simulink model "6DoF_V8_2024a_FULLY_WORKING_FG"  (R2024b)
settings: Solver=ode45  StartTime=0.0  StopTime=500  FixedStep=.01  MaxStep=.004  RelTol=1e-5  EnableMultiTasking=on
values from neighbouring files (symbols this model uses):
  ac = [0 0 0]    [Geom_6dof_V4_WITH_MAP.m]
  b = 33.4    [Geom_6dof_V4_WITH_MAP.m]
  bankrange = linspace(-pi,pi,100)    [Geom_6dof_V4_WITH_MAP.m]
  cbar = 5.7    [Geom_6dof_V4_WITH_MAP.m]
  cda2 = 0.33    [Geom_6dof_V4_WITH_MAP.m]
  cdo = 0.05    [Geom_6dof_V4_WITH_MAP.m]
  cg = [0 0 0]    [Geom_6dof_V4_WITH_MAP.m]
  cla = 4.44    [Geom_6dof_V4_WITH_MAP.m]
  cladot = 0    [Geom_6dof_V4_WITH_MAP.m]
  clb = -0.074    [Geom_6dof_V4_WITH_MAP.m]
  clda = -0.134    [Geom_6dof_V4_WITH_MAP.m]
  clde = 0.355    [Geom_6dof_V4_WITH_MAP.m]
  cldr = 0.107    [Geom_6dof_V4_WITH_MAP.m]
  clo = 0.41    [Geom_6dof_V4_WITH_MAP.m]
  clp = -0.410    (= -0.41)    [Geom_6dof_V4_WITH_MAP.m]
  clq = 3.8    [Geom_6dof_V4_WITH_MAP.m]
  clr = 0.107    [Geom_6dof_V4_WITH_MAP.m]
  cma = -0.683    [Geom_6dof_V4_WITH_MAP.m]
  cmadot = -4.36    [Geom_6dof_V4_WITH_MAP.m]
  cmde = -0.923    [Geom_6dof_V4_WITH_MAP.m]
  cmq = -9.96    [Geom_6dof_V4_WITH_MAP.m]
  cnb = 0.071    [Geom_6dof_V4_WITH_MAP.m]
  cnda = -0.0035    [Geom_6dof_V4_WITH_MAP.m]
  cndr = -0.072    [Geom_6dof_V4_WITH_MAP.m]
  cnp = -0.0575    [Geom_6dof_V4_WITH_MAP.m]
  cnr = -0.125    [Geom_6dof_V4_WITH_MAP.m]
  cyb = -0.564    [Geom_6dof_V4_WITH_MAP.m]
  cydr = 0.157    [Geom_6dof_V4_WITH_MAP.m]
  eng = [0 0 0]    [Geom_6dof_V4_WITH_MAP.m]
  initalt = 5000    [Geom_6dof_V4_WITH_MAP.m]
  initbank = 0    [Geom_6dof_V4_WITH_MAP.m]
  initeast = 0    [Geom_6dof_V4_WITH_MAP.m]
  inithead = 0    [Geom_6dof_V4_WITH_MAP.m]
  initnorth = 0    [Geom_6dof_V4_WITH_MAP.m]
  initp = 0    [Geom_6dof_V4_WITH_MAP.m]
  initpitch = initw/initu    (= -0.0287187462721)    [Geom_6dof_V4_WITH_MAP.m]
  initq = 0    [Geom_6dof_V4_WITH_MAP.m]
  initr = 0    [Geom_6dof_V4_WITH_MAP.m]
  initu = 226.333    [Geom_6dof_V4_WITH_MAP.m]
  initv = 0    [Geom_6dof_V4_WITH_MAP.m]
  initw = -6.5    [Geom_6dof_V4_WITH_MAP.m]
  jx = 1048    [Geom_6dof_V4_WITH_MAP.m]
  jxz = 0    [Geom_6dof_V4_WITH_MAP.m]
  jy = 3000    [Geom_6dof_V4_WITH_MAP.m]
  jz = 3500    [Geom_6dof_V4_WITH_MAP.m]
  sw = 184    [Geom_6dof_V4_WITH_MAP.m]
  weight = 2750    [Geom_6dof_V4_WITH_MAP.m]
  WP1 = [10000 10000 5000]    [Geom_6dof_V4_WITH_MAP.m]
  WP2 = [-10000 0 5500]    [Geom_6dof_V4_WITH_MAP.m]
  WP3 = [0 -10000 4500]    [Geom_6dof_V4_WITH_MAP.m]
libraries: slpidlib x10, simulink_extras x5, aerolibfltsims x2, aerolibanimutils x1, dspswit3 x1
(part 1 of 2)
settings Model: Creator=andersop  LastModifiedBy=Owner
settings SolverCC: InitialStep=.004  AlgebraicLoopSolver=TrustRegion
settings DataIOCC: LimitDataPoints=on  SaveFormat=Array  SignalLoggingSaveFormat=ModelDataLogs  SaveState=on  ReturnWorkspaceOutputs=off  SignalLoggingName=sigsOut
settings OptimizationCC: ExpressionDepthLimit=2147483647  InitFltsAndDblsToZero=on  LifeSpan=inf
settings DebuggingCC: SaveWithParameterizedLinksMsg=none  UnderspecifiedInitializationDetection=Classic  MergeDetectMultiDrivingBlocksExec=none  SignalResolutionControl=TryResolveAllWithWarning  MultiTaskDSMMsg=warning  MultiTaskCondExecSysMsg=none  FcnCallInpInsideContextMsg=warning  UnconnectedInputMsg=warning  UnconnectedOutputMsg=warning  UnconnectedLineMsg=warning  StateNameClashWarn=warning  SFUnexpectedBacktrackingDiag=warning  SFNoUnconditionalDefaultTransitionDiag=warning  SFExecutionAtInitializationDiag=none  ArithmeticOperatorsInVariantConditions=warning
settings HardwareCC: ProdBitPerPointer=32  ProdBitPerSizeT=32  ProdBitPerPtrDiffT=32  ProdLargestAtomicFloat=None  ProdIntDivRoundTo=Undefined  ProdEndianess=Unspecified  ProdWordSize=32  ProdHWDeviceType=32-bit Generic  TargetUnknown=on
settings ModelReferenceCC: PropagateSignalLabelsOutOfModel=off
settings SFSimCC: SimUseLocalCustomCode=off  CustomCodeUndefinedFunction=UseInterfaceOnly
settings RTWCC: RTWUseLocalCustomCode=off  GPUComputeCapability=3.5
settings CodeAppCC: StateflowObjectComments=on
settings GRTTargetCC: TargetFcnLib=ansi_tfl_tmw.mat  TargetLangStandard=C89/C90 (ANSI)  ModelReferenceCompliant=off  CombineOutputUpdateFcns=off  MatFileLogging=off  GRTInterface=on
settings ConfigComp: CovMetricSettings=dw  CovSaveCumulativeToWorkspaceVar=on  CovSaveSingleToWorkspaceVar=on  CovExternalEMLEnable=off

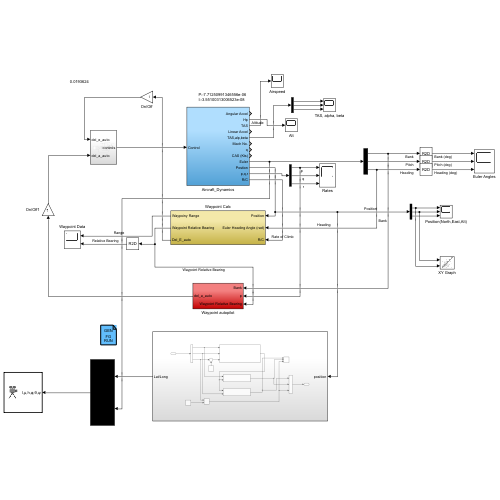
[thumbnail: Simulink's stored preview of the top-level diagram]
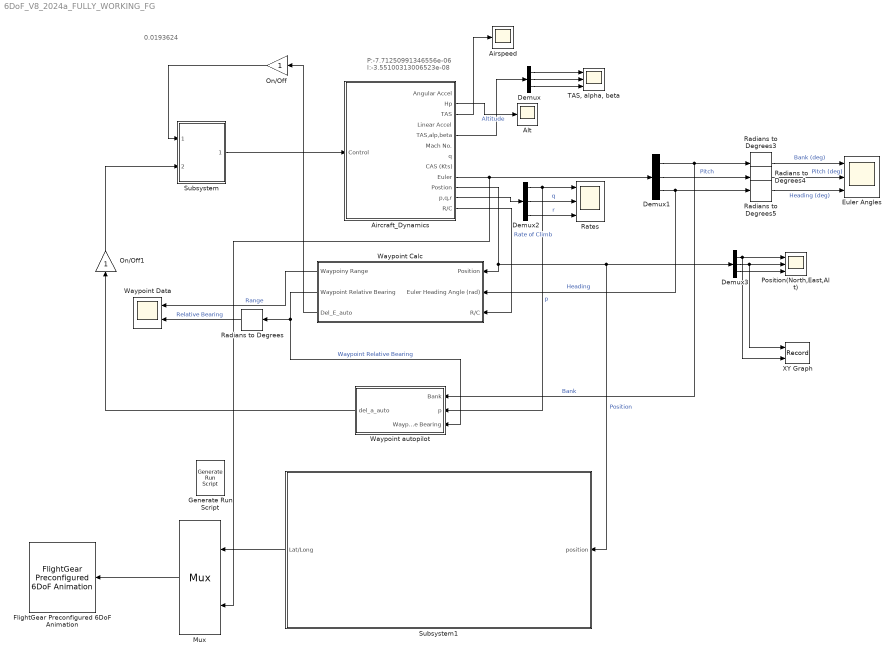
== system 6DoF_V8_2024a_FULLY_WORKING_FG ==
  note: P:-7.71250991346556e-06
      | I:-3.55100313006523e-08
  note: 0.0193624
  Aircraft_Dynamics : Subsystem
  Airspeed : Scope
  Alt : Scope
  Demux{,1..3} (4 alike) : Demux  Outputs=3
  Euler Angles : Scope  NumInputPorts=3
  FlightGear Preconfigured 6DoF Animation : aerolibfltsims/FlightGear Preconfigured 6DoF Animation  xFlightGearVersion=v2019.1  DestinationIpAddress=127.0.0.1  DestinationPort=5502  SampleTime=1/30  packetVersion=24
  Generate Run Script : aerolibfltsims/Generate Run Script  Architecture=Win64  dataFlow=Send  GeometryModelName=c172p  AirportId=KSFO  RunwayId=10L  InitialAltitude=5000  InitialHeading=0  OffsetDistance=4.72  OffsetAzimuth=0  InstallScenery=off  DisableShaders=off  OriginAddress=127.0.0.1  DestinationPort=5502  OriginPort=5505  LocalAddress=127.0.0.1  OutputFileName=runfg.bat  FlightGearBaseDirectory=C:\Program Files\FlightGear 2020.3
  Mux : Mux  Inputs=2
  On/Off : Gain
  On/Off1 : Gain
  Position(North,East,Alt) : Scope  NumInputPorts=3
  Radians to Degrees{,3..5} (4 alike) : simulink_extras/Transformations/Radians to Degrees
  Rates : Scope  NumInputPorts=3
  Subsystem : Subsystem
  Subsystem1 : Subsystem
  "TAS, alpha, beta" : Scope  NumInputPorts=3
  Waypoint Calc : Subsystem
  Waypoint Data : Scope  NumInputPorts=2
  Waypoint autopilot : Subsystem
  XY Graph : Record  FileSettingsInternal="{\"entries\":[{\"content\":{\"excelSettings\":{\"content\":{},\"type\":\"Streamout.ExcelSettings\"}},\"type\":\"Streamout.FileSettingStorage\",\"uuid\":\"\"}],\"packageUris\":[\"http:\\/\\/schema.mathworks.com\\/mf0\\/streamout_blocks\\/R2020a\"],\"version\":\"1.0\"}"  Layout=[1 1]  SignalsInternal="{\"entries\":[{\"content\":{\"signals\":[{\"content\":{\"blockPath\":[],\"dimensions\":[1],\"domain\":\"\",\"lineColor\":\"#a2142f\",\"plots\":[ 1 ],\"port\":1,\"sid\":[\"\"],\"signalID\":1,\"signalName\":\"Demux3:2\"},\"type\":\"RecordBlkView.Signal\",\"uuid\":\"\"},{\"content\":{\"blockPath\":[],\"dimensions\":[1],\"domain\":\"\",\"lineColor\":\"#139fff\",\"plots\":[ 1 ],\"port\":2,\"sid\":[\"\"],\"signalID\":2,\"signalName\":\"Demux3:1\"},\"type\":\"RecordBlkView.Signal\",\"uuid\":\"\"}]},\"type\":\"RecordBlkView.InputSignals\",\"uuid\":\"\"}],\"packageUris\":[\"http:\\/\\/schema.mathworks.com\\/mf0\\/streamout_blocks\\/R2020a\"],\"version\":\"1.0\"}"  VisualizationBindings="{\"xyplotplugin\":{\"info\":[{\"series\":[{\"bindingParametersList\":[{\"parameter\":\"X-Axis\",\"signalID\":1,\"signalName\":\"Demux3:2\"},{\"parameter\":\"Y-Axis\",\"signalID\":2,\"signalName\":\"Demux3:1\"}],\"seriesID\":0}],\"subplotID\":1}]}}"  CompatibilityTag=XY
  wires:
  Aircraft_Dynamics/9(Euler) -> Mux/2, Demux1/1
  Aircraft_Dynamics/3(TAS) -> Airspeed/1
  Aircraft_Dynamics/5(TAS,alp,beta) -> Demux/1
  Demux1/1 -> Waypoint autopilot/1(Bank), Radians to Degrees3/1  "Bank"
  Demux1/2 -> Radians to Degrees4/1  "Pitch"
  Demux1/3 -> Radians to Degrees5/1, Waypoint Calc/2(Euler Heading Angle (rad))  "Heading"
  Demux/1 -> "TAS, alpha, beta"/1
  Demux/2 -> "TAS, alpha, beta"/2
  Demux/3 -> "TAS, alpha, beta"/3
  Demux2/1 -> Rates/1, Waypoint autopilot/2(p)  "p"
  Demux2/2 -> Rates/2  "q"
  Demux2/3 -> Rates/3  "r"
  Aircraft_Dynamics/11(p,q,r) -> Demux2/1
  Aircraft_Dynamics/12(R/C) -> Waypoint Calc/3(R/C)  "Rate of Climb"
  Aircraft_Dynamics/10(Postion) -> Subsystem1/1(position), Demux3/1, Waypoint Calc/1(Position)  "Position"
  Demux3/1 -> XY Graph/2, Position(North,East,Alt)/1
  Demux3/2 -> XY Graph/1, Position(North,East,Alt)/2
  Demux3/3 -> Position(North,East,Alt)/3
  Waypoint Calc/1(Waypoiny Range) -> Waypoint Data/1  "Range"
  Waypoint Calc/2(Waypoint Relative Bearing) -> Radians to Degrees/1, Waypoint autopilot/3(Waypoint Relative Bearing)  "Waypoint Relative Bearing"
  Radians to Degrees/1 -> Waypoint Data/2  "Relative Bearing"
  Waypoint Calc/3(Del_E_auto) -> On/Off/1
  Radians to Degrees3/1 -> Euler Angles/1  "Bank (deg)"
  Radians to Degrees4/1 -> Euler Angles/2  "Pitch (deg)"
  Radians to Degrees5/1 -> Euler Angles/3  "Heading (deg)"
  Waypoint autopilot/1(del_a_auto) -> On/Off1/1
  Aircraft_Dynamics/2(Hp) -> Alt/1  "Altitude"
  Subsystem/1(controls) -> Aircraft_Dynamics/1(Control)
  On/Off/1 -> Subsystem/1(del_e_auto)
  On/Off1/1 -> Subsystem/2(del_a_auto)
  Subsystem1/1(Lat/Long) -> Mux/1
  Mux/1 -> FlightGear Preconfigured 6DoF Animation/1

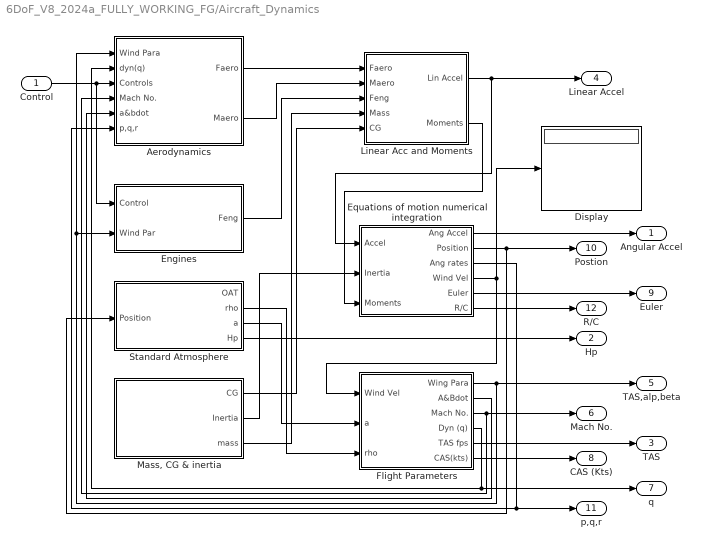
== system 6DoF_V8_2024a_FULLY_WORKING_FG/Aircraft_Dynamics ==
  Control : Inport
  Aerodynamics : Subsystem
  Display : Display
  Engines : Subsystem
  "Equations of motion numerical integration " : Subsystem
  Flight Parameters : Subsystem
  Linear Acc and Moments : Subsystem
  "Mass, CG & inertia" : Subsystem
  Standard Atmosphere : Subsystem
  Angular Accel : Outport
  Hp : Outport  Port=2
  TAS : Outport  Port=3
  Linear Accel : Outport  Port=4
  TAS,alp,beta : Outport  Port=5
  Mach No. : Outport  Port=6
  q : Outport  Port=7
  CAS (Kts) : Outport  Port=8
  Euler : Outport  Port=9
  Postion : Outport  Port=10
  p,q,r : Outport  Port=11
  R/C : Outport  Port=12
  wires:
  Aerodynamics/1(Faero) -> Linear Acc and Moments/1(Faero)
  Aerodynamics/2(Maero) -> Linear Acc and Moments/2(Maero)
  Control/1 -> Aerodynamics/3(Controls), Engines/1(Control)
  Engines/1(Feng) -> Linear Acc and Moments/3(Feng)
  "Mass, CG & inertia"/1(CG) -> Linear Acc and Moments/5(CG)
  "Mass, CG & inertia"/2(Inertia) -> "Equations of motion numerical integration "/2(Inertia)
  Linear Acc and Moments/1(Lin Accel) -> "Equations of motion numerical integration "/1(Accel), Linear Accel/1
  Linear Acc and Moments/2(Moments) -> "Equations of motion numerical integration "/3(Moments)
  "Equations of motion numerical integration "/3(Ang rates) -> Aerodynamics/6(p,q,r), p,q,r/1
  "Equations of motion numerical integration "/4(Wind Vel) -> Flight Parameters/1(Wind Vel), Display/1
  Flight Parameters/1(Wing Para) -> TAS,alp,beta/1, Aerodynamics/1(Wind Para), Engines/2(Wind Par)
  Flight Parameters/4(Dyn (q)) -> Aerodynamics/2(dyn(q)), q/1
  Flight Parameters/3(Mach No.) -> Mach No./1, Aerodynamics/4(Mach No.)
  Flight Parameters/2(A&Bdot) -> Aerodynamics/5(a&bdot)
  "Equations of motion numerical integration "/2(Position) -> Standard Atmosphere/1(Position), Postion/1
  "Equations of motion numerical integration "/1(Ang Accel) -> Angular Accel/1
  Standard Atmosphere/4(Hp) -> Hp/1
  Flight Parameters/5(TAS fps) -> TAS/1
  Flight Parameters/6(CAS(kts)) -> CAS (Kts)/1
  "Equations of motion numerical integration "/5(Euler) -> Euler/1
  Standard Atmosphere/3(a) -> Flight Parameters/2(a)
  Standard Atmosphere/2(rho) -> Flight Parameters/3(rho)
  "Mass, CG & inertia"/3(mass) -> Linear Acc and Moments/4(Mass)
  "Equations of motion numerical integration "/6(R/C) -> R/C/1

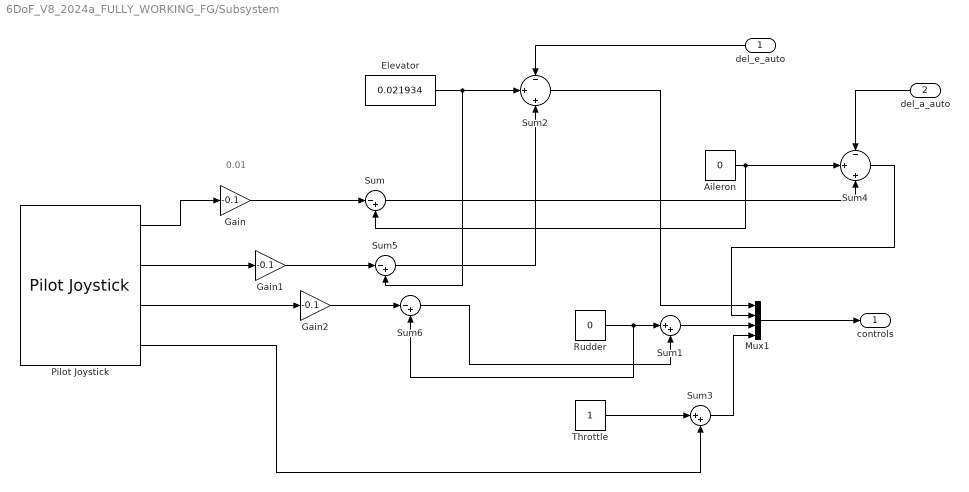
== system 6DoF_V8_2024a_FULLY_WORKING_FG/Subsystem ==
  note: 0.01
  del_e_auto : Inport
  del_a_auto : Inport  Port=2
  Aileron : Constant  Value=0
  Elevator : Constant  Value=0.021934
  Gain : Gain  Gain=-0.1
  Gain1 : Gain  Gain=-0.1
  Gain2 : Gain  Gain=-0.1
  Mux1 : Mux
  Pilot Joystick : aerolibanimutils/Pilot Joystick  JoystickID=Joystick1  OutputConfiguration=FourAxis  SampleTime=1/30
  Rudder : Constant  Value=0
  Sum : Sum  Inputs=|-+
  Sum1 : Sum  Inputs=|++
  Sum2 : Sum  Inputs=-|+|+
  Sum3 : Sum  Inputs=|++
  Sum4 : Sum  Inputs=-|+|+
  Sum5 : Sum  Inputs=|-+
  Sum6 : Sum  Inputs=|-+
  Throttle : Constant
  controls : Outport
  wires:
  Elevator/1 -> Sum2/2, Sum5/2
  Pilot Joystick/1 -> Gain/1
  Gain1/1 -> Sum5/1
  Pilot Joystick/3 -> Gain2/1
  Sum2/1 -> Mux1/1
  Sum4/1 -> Mux1/2
  Pilot Joystick/2 -> Gain1/1
  Gain2/1 -> Sum6/1
  Sum5/1 -> Sum2/3
  Gain/1 -> Sum/1
  Mux1/1 -> controls/1
  del_e_auto/1 -> Sum2/1
  Aileron/1 -> Sum4/2, Sum/2
  Sum/1 -> Sum4/3
  del_a_auto/1 -> Sum4/1
  Rudder/1 -> Sum6/2, Sum1/1
  Sum6/1 -> Sum1/2
  Sum1/1 -> Mux1/3
  Throttle/1 -> Sum3/1
  Pilot Joystick/4 -> Sum3/2
  Sum3/1 -> Mux1/4

== system 6DoF_V8_2024a_FULLY_WORKING_FG/Subsystem1 ==
  position : Inport
  Demux : Demux  Outputs=3
  Earth : Constant  Value=20925000
  MATLAB Function : MATLAB Function  TreatAsAtomicUnit=on
  MATLAB Function1 : MATLAB Function  TreatAsAtomicUnit=on
  Mux : Mux  Inputs=3
  "NED to LAT/LONG " : Subsystem
  Product : Product
  Scope : Scope  NumInputPorts=3
  Sum : Sum  Inputs=|++
  ft - m conversion : Constant  Value=0.3048
  Lat/Long : Outport
  wires:
  Mux/1 -> Lat/Long/1
  Demux/3 -> Product/1, Sum/1
  Demux/1 -> MATLAB Function/1(N), "NED to LAT/LONG "/1(N)
  "NED to LAT/LONG "/1(r) -> MATLAB Function1/1(r), MATLAB Function/2(r)
  MATLAB Function/1(Lat) -> Mux/2, Scope/2
  Demux/2 -> MATLAB Function1/2(E), "NED to LAT/LONG "/2(E)
  Sum/1 -> "NED to LAT/LONG "/3(D)
  position/1 -> Demux/1
  Earth/1 -> Sum/2
  MATLAB Function1/1(Long) -> Mux/1, Scope/1
  Product/1 -> Mux/3, Scope/3
  ft - m conversion/1 -> Product/2

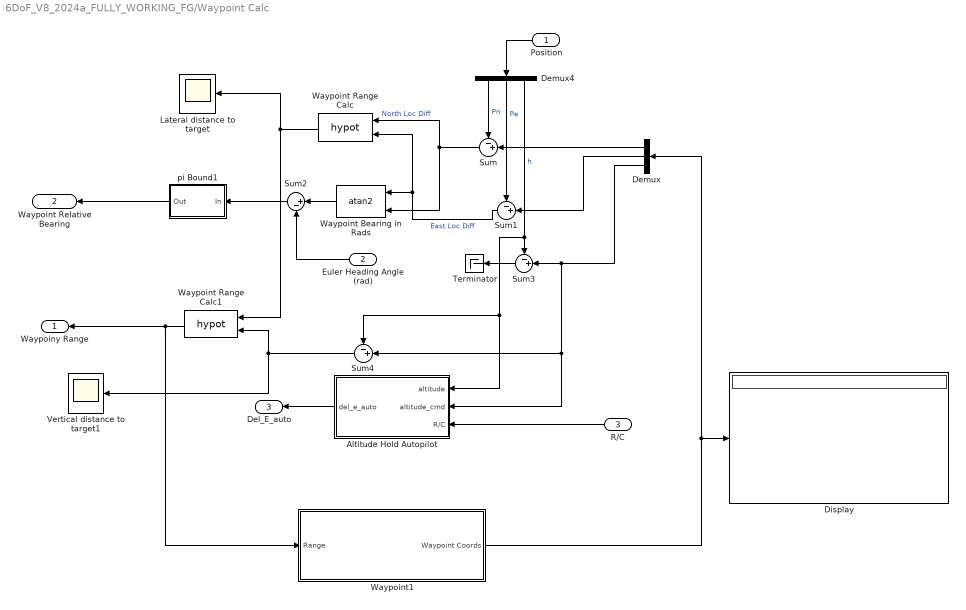
== system 6DoF_V8_2024a_FULLY_WORKING_FG/Waypoint Calc ==
  Position : Inport
  Euler Heading Angle (rad) : Inport  Port=2
  R/C : Inport  Port=3
  Altitude Hold Autopilot : Subsystem
  Demux : Demux  Outputs=3
  Demux4 : Demux  Outputs=3
  Display : Display
  Lateral distance to target : Scope
  Sum{,1,3..4} (4 alike) : Sum  Inputs=-+|
  Sum2 : Sum  Inputs=|+-
  Terminator : Terminator
  Vertical distance to target1 : Scope
  Waypoint Bearing in Rads : Trigonometry  Operator=atan2
  Waypoint Range Calc : Math  Operator=hypot
  Waypoint Range Calc1 : Math  Operator=hypot
  Waypoint1 : Subsystem
  pi Bound1 : Subsystem  mask(pi bound){}
      mask help: Bounds the input angle to [-pi, pi]. When -pi bound is exceeded the output wraps back to pi; when the pi bound is exceeded the output wraps back to -pi.
      mask Help:
      | Bounds the input angle to [-pi, pi]. When -pi bound is exceeded the output wraps back to pi; when the pi bound is exceeded the output wraps back to -pi.
      | <P><B>Input:</B> any angle in radians, from -Inf to Inf;</P>
      | <P><B>Output:</B> an angle in radians between -pi and pi.</P>
  Waypoiny Range : Outport
  Waypoint Relative Bearing : Outport  Port=2
  Del_E_auto : Outport  Port=3
  wires:
  Demux4/2 -> Sum1/1  "Pe"
  Sum/1 -> Waypoint Bearing in Rads/2, Waypoint Range Calc/1  "North Loc Diff"
  Demux4/3 -> Sum4/1, Altitude Hold Autopilot/1(altitude), Sum3/1  "h"
  Sum1/1 -> Waypoint Bearing in Rads/1, Waypoint Range Calc/2  "East Loc Diff"
  Sum3/1 -> Terminator/1
  Demux4/1 -> Sum/1  "Pn"
  Position/1 -> Demux4/1
  Waypoint Range Calc/1 -> Lateral distance to target/1, Waypoint Range Calc1/1
  Euler Heading Angle (rad)/1 -> Sum2/2
  Waypoint Bearing in Rads/1 -> Sum2/1
  Sum2/1 -> pi Bound1/1(In)
  pi Bound1/1(Out) -> Waypoint Relative Bearing/1
  Demux/1 -> Sum/2
  Demux/2 -> Sum1/2
  Demux/3 -> Altitude Hold Autopilot/2(altitude_cmd), Sum4/2, Sum3/2
  R/C/1 -> Altitude Hold Autopilot/3(R/C)
  Sum4/1 -> Vertical distance to target1/1, Waypoint Range Calc1/2
  Waypoint Range Calc1/1 -> Waypoint1/1(Range), Waypoiny Range/1
  Altitude Hold Autopilot/1(del_e_auto) -> Del_E_auto/1
  Waypoint1/1(Waypoint Coords) -> Demux/1, Display/1

== system 6DoF_V8_2024a_FULLY_WORKING_FG/Waypoint autopilot ==
  Bank : Inport
  p : Inport  Port=2
  Waypoint Relative Bearing : Inport  Port=3
  1 : slpidlib/PID Controller  Controller=PI  Form=Parallel  TimeDomain=Continuous-time  UseExternalTs=off  SampleTime=-1  IntegratorMethod=Forward Euler  FilterMethod=Forward Euler  ControllerParametersSource=internal  P=0.0442231432191756  I=0.000555878552542947  UseKiTs=off  D=-0.00015961532293143  UseExternalDerivativeSource=off  N=22.9108316729658  UseFilter=on  TunerSelectOption=Transfer Function Based (PID Tuner App)  InitialConditionSource=internal  InitialConditionForIntegrator=0  InitialConditionForFilter=0  DifferentiatorICPrevScaledInput=0  ExternalReset=none  TrackingMode=off  Kt=1  LimitOutput=off  SatLimitsSource=internal  UpperSaturationLimit=inf  LowerSaturationLimit=-inf  LinearizeAsGain=on  AntiWindupMode=none  Kb=1  LimitIntegrator=off  UpperIntegratorSaturationLimit=inf  LowerIntegratorSaturationLimit=-inf  POutMin=[]  POutMax=[]  IOutMin=[]  IOutMax=[]  DOutMin=[]  DOutMax=[]  NOutMin=[]  NOutMax=[]  SumOutMin=[]  SumOutMax=[]  SaturationOutMin=[]  SaturationOutMax=[]  PParamMin=[]  PParamMax=[]  IParamMin=[]  IParamMax=[]  DParamMin=[]  DParamMax=[]  NParamMin=[]  NParamMax=[]  KbParamMin=[]  KbParamMax=[]  KtParamMin=[]  KtParamMax=[]  KbOutMin=[]  KbOutMax=[]  KtOutMin=[]  KtOutMax=[]  IntegratorOutMin=[]  IntegratorOutMax=[]  FilterOutMin=[]  FilterOutMax=[]  SumI1OutMin=[]  SumI1OutMax=[]  SumI2OutMin=[]  SumI2OutMax=[]  SumI3OutMin=[]  SumI3OutMax=[]  SumI4OutMin=[]  SumI4OutMax=[]  SumDOutMin=[]  SumDOutMax=[]  DifferentiatorOutMin=[]  DifferentiatorOutMax=[]  FilterDiffOutCoefMin=[]  FilterDiffOutCoefMax=[]  ReciprocalOutMin=[]  ReciprocalOutMax=[]  SumDenOutMin=[]  SumDenOutMax=[]  SumNumOutMin=[]  SumNumOutMax=[]  DivideOutMin=[]  DivideOutMax=[]  UdiffTsProdOutMin=[]  UdiffTsProdOutMax=[]  NTsProdOutMin=[]  NTsProdOutMax=[]  UintegralTsProdOutMin=[]  UintegralTsProdOutMax=[]  UngainTsProdOutMin=[]  UngainTsProdOutMax=[]  ClampingZeroOutDataTypeStr=Inherit: Inherit via back propagation  ClampingZeroOutMin=[]  ClampingZeroOutMax=[]  FilterDenConstantOutDataTypeStr=Inherit: Inherit via back propagation  FilterDenConstantOutMin=[]  FilterDenConstantOutMax=[]  PCopyOutDataTypeStr=Inherit: Inherit via back propagation  PCopyOutMin=[]  PCopyOutMax=[]  NCopyOutDataTypeStr=Inherit: Inherit via back propagation  NCopyOutMin=[]  NCopyOutMax=[]  IntegratorContinuousStateAttributes=''  IntegratorStateMustResolveToSignalObject=off  IntegratorRTWStateStorageClass=Auto  FilterContinuousStateAttributes=''  FilterStateMustResolveToSignalObject=off  FilterRTWStateStorageClass=Auto  ParallelPVariant=InternalParameters  IdealPVariant=Disabled  IVariant=InternalParameters  DVariant=Disabled  IntegratorVariant=Continuous  SatVariant=Disabled  AWVariant=Passthrough  PCopyVariant=Disabled  TRVariant=Disabled  FdbkBlocksVariant=Forward  IdealPFdbkVariant=Disabled  SatFdbkVariant=Disabled  DerivativeFilterVariant=Disabled  NVariant=Disabled  NCopyVariant=Disabled_SignalSpec  FilterICVariant=Disabled  IntegratorICVariant=InternalICs  ExternalResetVariant=Disabled  TRSumVariant=Passthrough  SumFdbkVariant=Disabled  SumVariant=Sum_PI  TsampFilterVariant=InternalTs  TsampNgainVariant=Passthrough  TsampIntegralVariant=Disabled_SignalSpec  ExternalSaturationOutDataTypeStr=Inherit: Same as second input  DerivativeSourceVariant=Disabled  PreIntVariant=InternalPreInt
  2 : slpidlib/PID Controller  Controller=PI  Form=Parallel  TimeDomain=Continuous-time  UseExternalTs=off  SampleTime=-1  IntegratorMethod=Forward Euler  FilterMethod=Forward Euler  ControllerParametersSource=internal  P=0.0813778181648477  I=0.00542773234625677  UseKiTs=off  D=-0.00015961532293143  UseExternalDerivativeSource=off  N=22.9108316729658  UseFilter=on  TunerSelectOption=Transfer Function Based (PID Tuner App)  InitialConditionSource=internal  InitialConditionForIntegrator=0  InitialConditionForFilter=0  DifferentiatorICPrevScaledInput=0  ExternalReset=none  TrackingMode=off  Kt=1  LimitOutput=off  SatLimitsSource=internal  UpperSaturationLimit=inf  LowerSaturationLimit=-inf  LinearizeAsGain=on  AntiWindupMode=none  Kb=1  LimitIntegrator=off  UpperIntegratorSaturationLimit=inf  LowerIntegratorSaturationLimit=-inf  POutMin=[]  POutMax=[]  IOutMin=[]  IOutMax=[]  DOutMin=[]  DOutMax=[]  NOutMin=[]  NOutMax=[]  SumOutMin=[]  SumOutMax=[]  SaturationOutMin=[]  SaturationOutMax=[]  PParamMin=[]  PParamMax=[]  IParamMin=[]  IParamMax=[]  DParamMin=[]  DParamMax=[]  NParamMin=[]  NParamMax=[]  KbParamMin=[]  KbParamMax=[]  KtParamMin=[]  KtParamMax=[]  KbOutMin=[]  KbOutMax=[]  KtOutMin=[]  KtOutMax=[]  IntegratorOutMin=[]  IntegratorOutMax=[]  FilterOutMin=[]  FilterOutMax=[]  SumI1OutMin=[]  SumI1OutMax=[]  SumI2OutMin=[]  SumI2OutMax=[]  SumI3OutMin=[]  SumI3OutMax=[]  SumI4OutMin=[]  SumI4OutMax=[]  SumDOutMin=[]  SumDOutMax=[]  DifferentiatorOutMin=[]  DifferentiatorOutMax=[]  FilterDiffOutCoefMin=[]  FilterDiffOutCoefMax=[]  ReciprocalOutMin=[]  ReciprocalOutMax=[]  SumDenOutMin=[]  SumDenOutMax=[]  SumNumOutMin=[]  SumNumOutMax=[]  DivideOutMin=[]  DivideOutMax=[]  UdiffTsProdOutMin=[]  UdiffTsProdOutMax=[]  NTsProdOutMin=[]  NTsProdOutMax=[]  UintegralTsProdOutMin=[]  UintegralTsProdOutMax=[]  UngainTsProdOutMin=[]  UngainTsProdOutMax=[]  ClampingZeroOutDataTypeStr=Inherit: Inherit via back propagation  ClampingZeroOutMin=[]  ClampingZeroOutMax=[]  FilterDenConstantOutDataTypeStr=Inherit: Inherit via back propagation  FilterDenConstantOutMin=[]  FilterDenConstantOutMax=[]  PCopyOutDataTypeStr=Inherit: Inherit via back propagation  PCopyOutMin=[]  PCopyOutMax=[]  NCopyOutDataTypeStr=Inherit: Inherit via back propagation  NCopyOutMin=[]  NCopyOutMax=[]  IntegratorContinuousStateAttributes=''  IntegratorStateMustResolveToSignalObject=off  IntegratorRTWStateStorageClass=Auto  FilterContinuousStateAttributes=''  FilterStateMustResolveToSignalObject=off  FilterRTWStateStorageClass=Auto  ParallelPVariant=InternalParameters  IdealPVariant=Disabled  IVariant=InternalParameters  DVariant=Disabled  IntegratorVariant=Continuous  SatVariant=Disabled  AWVariant=Passthrough  PCopyVariant=Disabled  TRVariant=Disabled  FdbkBlocksVariant=Forward  IdealPFdbkVariant=Disabled  SatFdbkVariant=Disabled  DerivativeFilterVariant=Disabled  NVariant=Disabled  NCopyVariant=Disabled_SignalSpec  FilterICVariant=Disabled  IntegratorICVariant=InternalICs  ExternalResetVariant=Disabled  TRSumVariant=Passthrough  SumFdbkVariant=Disabled  SumVariant=Sum_PI  TsampFilterVariant=InternalTs  TsampNgainVariant=Passthrough  TsampIntegralVariant=Disabled_SignalSpec  ExternalSaturationOutDataTypeStr=Inherit: Same as second input  DerivativeSourceVariant=Disabled  PreIntVariant=InternalPreInt
  Bank Err : Scope
  Bearing Lookup1 : Lookup_n-D  NumberOfTableDimensions=1  BreakpointsForDimension1=bankrange  BreakpointsForDimension1Spacing=30  Table=(1.5/pi)*atan(bankrange)  InternalRulePriority=Speed  RndMeth=Simplest
  Del_a : Scope
  Orig : slpidlib/PID Controller  Controller=PI  Form=Parallel  TimeDomain=Continuous-time  UseExternalTs=off  SampleTime=-1  IntegratorMethod=Forward Euler  FilterMethod=Forward Euler  ControllerParametersSource=internal  P=0.0584144917265337 *2.63  I=0.0031457168401691*0.57  UseKiTs=off  D=0  UseExternalDerivativeSource=off  N=100  UseFilter=on  TunerSelectOption=Transfer Function Based (PID Tuner App)  InitialConditionSource=internal  InitialConditionForIntegrator=0  InitialConditionForFilter=0  DifferentiatorICPrevScaledInput=0  ExternalReset=none  TrackingMode=off  Kt=1  LimitOutput=off  SatLimitsSource=internal  UpperSaturationLimit=inf  LowerSaturationLimit=-inf  LinearizeAsGain=on  AntiWindupMode=none  Kb=1  LimitIntegrator=off  UpperIntegratorSaturationLimit=inf  LowerIntegratorSaturationLimit=-inf  POutMin=[]  POutMax=[]  IOutMin=[]  IOutMax=[]  DOutMin=[]  DOutMax=[]  NOutMin=[]  NOutMax=[]  SumOutMin=[]  SumOutMax=[]  SaturationOutMin=[]  SaturationOutMax=[]  PParamMin=[]  PParamMax=[]  IParamMin=[]  IParamMax=[]  DParamMin=[]  DParamMax=[]  NParamMin=[]  NParamMax=[]  KbParamMin=[]  KbParamMax=[]  KtParamMin=[]  KtParamMax=[]  KbOutMin=[]  KbOutMax=[]  KtOutMin=[]  KtOutMax=[]  IntegratorOutMin=[]  IntegratorOutMax=[]  FilterOutMin=[]  FilterOutMax=[]  SumI1OutMin=[]  SumI1OutMax=[]  SumI2OutMin=[]  SumI2OutMax=[]  SumI3OutMin=[]  SumI3OutMax=[]  SumI4OutMin=[]  SumI4OutMax=[]  SumDOutMin=[]  SumDOutMax=[]  DifferentiatorOutMin=[]  DifferentiatorOutMax=[]  FilterDiffOutCoefMin=[]  FilterDiffOutCoefMax=[]  ReciprocalOutMin=[]  ReciprocalOutMax=[]  SumDenOutMin=[]  SumDenOutMax=[]  SumNumOutMin=[]  SumNumOutMax=[]  DivideOutMin=[]  DivideOutMax=[]  UdiffTsProdOutMin=[]  UdiffTsProdOutMax=[]  NTsProdOutMin=[]  NTsProdOutMax=[]  UintegralTsProdOutMin=[]  UintegralTsProdOutMax=[]  UngainTsProdOutMin=[]  UngainTsProdOutMax=[]  ClampingZeroOutDataTypeStr=Inherit: Inherit via back propagation  ClampingZeroOutMin=[]  ClampingZeroOutMax=[]  FilterDenConstantOutDataTypeStr=Inherit: Inherit via back propagation  FilterDenConstantOutMin=[]  FilterDenConstantOutMax=[]  PCopyOutDataTypeStr=Inherit: Inherit via back propagation  PCopyOutMin=[]  PCopyOutMax=[]  NCopyOutDataTypeStr=Inherit: Inherit via back propagation  NCopyOutMin=[]  NCopyOutMax=[]  IntegratorContinuousStateAttributes=''  IntegratorStateMustResolveToSignalObject=off  IntegratorRTWStateStorageClass=Auto  FilterContinuousStateAttributes=''  FilterStateMustResolveToSignalObject=off  FilterRTWStateStorageClass=Auto  ParallelPVariant=InternalParameters  IdealPVariant=Disabled  IVariant=InternalParameters  DVariant=Disabled  IntegratorVariant=Continuous  SatVariant=Disabled  AWVariant=Passthrough  PCopyVariant=Disabled  TRVariant=Disabled  FdbkBlocksVariant=Forward  IdealPFdbkVariant=Disabled  SatFdbkVariant=Disabled  DerivativeFilterVariant=Disabled  NVariant=Disabled  NCopyVariant=Disabled_SignalSpec  FilterICVariant=Disabled  IntegratorICVariant=InternalICs  ExternalResetVariant=Disabled  TRSumVariant=Passthrough  SumFdbkVariant=Disabled  SumVariant=Sum_PI  TsampFilterVariant=InternalTs  TsampNgainVariant=Passthrough  TsampIntegralVariant=Disabled_SignalSpec  ExternalSaturationOutDataTypeStr=Inherit: Same as second input  DerivativeSourceVariant=Disabled  PreIntVariant=InternalPreInt
  P Desired : Scope
  Radians to Degrees1 : simulink_extras/Transformations/Radians to Degrees
  Sum1 : Sum  Inputs=+|-
  Sum3 : Sum  Inputs=+|-
  p Lookup : Lookup_n-D  NumberOfTableDimensions=1  BreakpointsForDimension1=bankrange  BreakpointsForDimension1Spacing=30  Table=0.18*atan(bankrange)  InternalRulePriority=Speed  RndMeth=Simplest
  perr : Scope
  del_a_auto : Outport
  wires:
  Bearing Lookup1/1 -> Sum1/2  "Bank Desired"
  Radians to Degrees1/1 -> Bank Err/1
  Sum1/1 -> Radians to Degrees1/1, p Lookup/1
  Sum3/1 -> Orig/1, perr/1  "Perr"
  Bank/1 -> Sum1/1
  p Lookup/1 -> P Desired/1, Sum3/2  "P Desired"
  Waypoint Relative Bearing/1 -> Bearing Lookup1/1
  p/1 -> Sum3/1
  Orig/1 -> del_a_auto/1

== system 6DoF_V8_2024a_FULLY_WORKING_FG/Aircraft_Dynamics/Aerodynamics ==
  note: Notes: alpha is measured from
  Wind Para : Inport
  dyn(q) : Inport  Port=2
  Controls : Inport  Port=3
  Mach No. : Inport  Port=4
  a&bdot : Inport  Port=5
  p,q,r : Inport  Port=6
  Aero Forces and Moments : Subsystem
  CD : Subsystem
  CL : Subsystem
  CM : Subsystem
  CN : Subsystem
  CY : Subsystem
  Croll : Subsystem
  Faero : Outport
  Maero : Outport  Port=2
  wires:
  Wind Para/1 -> CY/1(Wind Parameters), Aero Forces and Moments/5(Wind Para), CN/1(Wind Parameters), Croll/1(Wind Parameters), CM/1(Wind Parameters), CD/1(Wind Parameters), CL/1(Wind Parameters)
  CL/1(CL) -> Aero Forces and Moments/4(CL)
  Mach No./1 -> CM/3(Mach No.), CN/3(Mach No.), Croll/3(Mach No.), CY/3(Mach No.), CL/3(Mach No.), CD/3(Mach No.)
  a&bdot/1 -> CL/4(a&bdot), CM/4(a&bdot)
  p,q,r/1 -> CM/5(P,q,r), CN/4(P,q,r), Croll/4(P,q,r), CY/4(P,q,r), CL/5(P,q,r)
  Controls/1 -> CM/2(Controls), CD/2(Controls), CN/2(Controls), Croll/2(Controls), CY/2(Controls), CL/2(Controls)
  CD/1(CD) -> Aero Forces and Moments/2(CD)
  CN/1(CN) -> Aero Forces and Moments/8(CN)
  Croll/1(Croll) -> Aero Forces and Moments/6(Croll)
  CY/1(CY) -> Aero Forces and Moments/3(CY)
  CM/1(CM) -> Aero Forces and Moments/7(CM)
  dyn(q)/1 -> Aero Forces and Moments/1(dyn(q))
  Aero Forces and Moments/1(Faero) -> Faero/1
  Aero Forces and Moments/2(Maero) -> Maero/1

== system 6DoF_V8_2024a_FULLY_WORKING_FG/Aircraft_Dynamics/Engines ==
  Control : Inport
  Wind Par : Inport  Port=2
  Demux : Demux
  Demux1 : Demux  Outputs=3
  Display : Display
  Max Power : Constant  Value=200*550
  Product : Product  RndMeth=Zero
  Product1 : Product  Inputs=*/  RndMeth=Zero
  Terminator{,1..4} (5 alike) : Terminator
  Feng : Outport
  wires:
  Max Power/1 -> Product/2
  Control/1 -> Demux/1
  Demux/4 -> Product/1
  Demux/1 -> Terminator/1
  Demux/2 -> Terminator1/1
  Demux/3 -> Terminator2/1
  Product/1 -> Product1/1
  Product1/1 -> Feng/1, Display/1
  Wind Par/1 -> Demux1/1
  Demux1/1 -> Product1/2
  Demux1/2 -> Terminator4/1
  Demux1/3 -> Terminator3/1

== system 6DoF_V8_2024a_FULLY_WORKING_FG/Aircraft_Dynamics/Equations of motion numerical integration  ==
  Accel : Inport
  Inertia : Inport  Port=2
  Moments : Inport  Port=3
  Flat Earth Navigation : Subsystem
  Force Equations : Subsystem
  Gravity Model : Subsystem
  Inert-body : Subsystem
  Kinematic Equiations : Subsystem
  Moment Equations : Subsystem
  Ang Accel : Outport
  Position : Outport  Port=2
  Ang rates : Outport  Port=3
  Wind Vel : Outport  Port=4
  Euler : Outport  Port=5
  R/C : Outport  Port=6
  wires:
  Moment Equations/1(Ang Rates) -> Kinematic Equiations/1(Rates), Force Equations/3(Rates), Ang rates/1
  Kinematic Equiations/1(Euler angles) -> Flat Earth Navigation/1(Euler Angles), Inert-body/1(Euler), Euler/1
  Force Equations/1(Lin Vel) -> Wind Vel/1, Flat Earth Navigation/2(Velocity)
  Accel/1 -> Force Equations/1(Accel)
  Inertia/1 -> Moment Equations/1(Inertia)
  Gravity Model/1(Gravity) -> Force Equations/2(Gravity)
  Moments/1 -> Moment Equations/2(Moments)
  Moment Equations/2(Ang Accel) -> Ang Accel/1
  Flat Earth Navigation/1(Position) -> Position/1
  Inert-body/1(NEDtoBC) -> Force Equations/4(NEDtoABC)
  Flat Earth Navigation/2(R/C) -> R/C/1

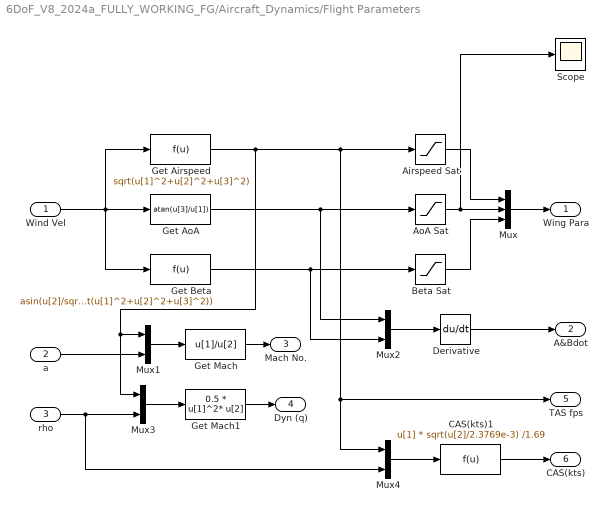
== system 6DoF_V8_2024a_FULLY_WORKING_FG/Aircraft_Dynamics/Flight Parameters ==
  Wind Vel : Inport
  a : Inport  Port=2
  rho : Inport  Port=3
  Airspeed Sat : Saturate  UpperLimit=1100  LowerLimit=0
  AoA Sat : Saturate  UpperLimit=0.3  LowerLimit=-0.2
  Beta Sat : Saturate  UpperLimit=0.4  LowerLimit=-0.4
  CAS(kts)1 : Fcn  Expr=u[1] * sqrt(u[2]/2.3769e-3) /1.69
  Derivative : Derivative
  Get Airspeed : Fcn  Expr=sqrt(u[1]^2+u[2]^2+u[3]^2)
  Get AoA : Fcn  Expr=atan(u[3]/u[1])
  Get Beta : Fcn  Expr=asin(u[2]/sqrt(u[1]^2+u[2]^2+u[3]^2))
  Get Mach : Fcn  Expr=u[1]/u[2]
  Get Mach1 : Fcn  Expr=0.5 * u[1]^2* u[2]
  Mux : Mux  Inputs=3
  Mux{1..4} (4 alike) : Mux  Inputs=2
  Scope : Scope
  Wing Para : Outport
  A&Bdot : Outport  Port=2
  Mach No. : Outport  Port=3
  Dyn (q) : Outport  Port=4
  TAS fps : Outport  Port=5
  CAS(kts) : Outport  Port=6
  wires:
  Wind Vel/1 -> Get AoA/1, Get Airspeed/1, Get Beta/1
  Get Airspeed/1 -> Mux1/1, Mux3/1, Airspeed Sat/1, TAS fps/1, Mux4/1
  Get AoA/1 -> AoA Sat/1, Mux2/1
  Get Beta/1 -> Beta Sat/1, Mux2/2
  AoA Sat/1 -> Mux/2, Scope/1
  Airspeed Sat/1 -> Mux/1
  Beta Sat/1 -> Mux/3
  Mux/1 -> Wing Para/1
  Mux1/1 -> Get Mach/1
  a/1 -> Mux1/2
  Mux2/1 -> Derivative/1
  Derivative/1 -> A&Bdot/1
  Get Mach/1 -> Mach No./1
  rho/1 -> Mux3/2, Mux4/2
  Mux3/1 -> Get Mach1/1
  Get Mach1/1 -> Dyn (q)/1
  Mux4/1 -> CAS(kts)1/1
  CAS(kts)1/1 -> CAS(kts)/1

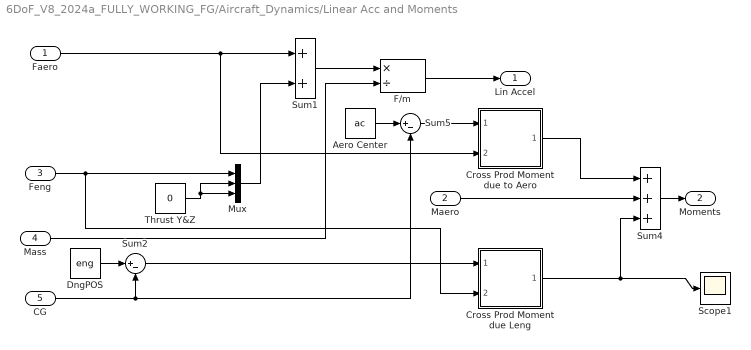
== system 6DoF_V8_2024a_FULLY_WORKING_FG/Aircraft_Dynamics/Linear Acc and Moments ==
  Faero : Inport
  Maero : Inport  Port=2
  Feng : Inport  Port=3
  Mass : Inport  Port=4
  CG : Inport  Port=5
  Aero Center : Constant  Value=ac
  Cross Prod Moment due Leng : Subsystem
  Cross Prod Moment due to Aero : Subsystem
  DngPOS : Constant  Value=eng
  F/m : Product  Inputs=*/  SaturateOnIntegerOverflow=on  OutDataTypeStr=Inherit: Same as first input
  Mux : Mux  Inputs=3
  Scope1 : Scope
  Sum1 : Sum  SaturateOnIntegerOverflow=on
  Sum2 : Sum  Inputs=|+-  SaturateOnIntegerOverflow=on
  Sum4 : Sum  Inputs=+++  SaturateOnIntegerOverflow=on
  Sum5 : Sum  Inputs=|+-  SaturateOnIntegerOverflow=on
  Thrust Y&Z : Constant  Value=0
  Lin Accel : Outport
  Moments : Outport  Port=2
  wires:
  Feng/1 -> Cross Prod Moment due Leng/2(Vec 2), Mux/1
  Thrust Y&Z/1 -> Mux/2, Mux/3
  Faero/1 -> Sum1/1, Cross Prod Moment due to Aero/2(Vec 2)
  Mux/1 -> Sum1/2
  Sum1/1 -> F/m/1
  Mass/1 -> F/m/2
  F/m/1 -> Lin Accel/1
  CG/1 -> Sum2/2, Sum5/2
  Aero Center/1 -> Sum5/1
  Sum5/1 -> Cross Prod Moment due to Aero/1(Vec 1)
  Maero/1 -> Sum4/2
  Sum4/1 -> Moments/1
  Cross Prod Moment due to Aero/1(X Prod) -> Sum4/1
  Sum2/1 -> Cross Prod Moment due Leng/1(Vec 1)
  Cross Prod Moment due Leng/1(X Prod) -> Sum4/3, Scope1/1
  DngPOS/1 -> Sum2/1

== system 6DoF_V8_2024a_FULLY_WORKING_FG/Aircraft_Dynamics/Mass, CG & inertia ==
  Mux1 : Mux
  cg : Constant  Value=cg
  jx : Constant  Value=jx
  jxz : Constant  Value=jxz
  jy : Constant  Value=jy
  jz : Constant  Value=jz
  mass2 : Constant  Value=weight/32.2
  CG : Outport
  Inertia : Outport  Port=2
  mass : Outport  Port=3
  wires:
  cg/1 -> CG/1
  jy/1 -> Mux1/2
  jx/1 -> Mux1/1
  jz/1 -> Mux1/3
  jxz/1 -> Mux1/4
  Mux1/1 -> Inertia/1
  mass2/1 -> mass/1

== system 6DoF_V8_2024a_FULLY_WORKING_FG/Aircraft_Dynamics/Standard Atmosphere ==
  Position : Inport
  Demux : Demux  Outputs=3
      settings: DisplayOption=none
  Density : Fcn  Expr=2.3769e-3*(1 - 0.703e-5 * u[1])^4.14
  OATemp : Lookup  InputValues=[0 35000 60000]  Table=[519 390 390]
  Speed of Sound : Fcn  Expr=sqrt(1.4*1716.3*u[1])
  Terminator : Terminator
  Terminator1 : Terminator
  OAT : Outport
  rho : Outport  Port=2
  a : Outport  Port=3
  Hp : Outport  Port=4
  wires:
  OATemp/1 -> OAT/1, Speed of Sound/1
  Density/1 -> rho/1
  Speed of Sound/1 -> a/1
  Position/1 -> Demux/1
  Demux/1 -> Terminator/1
  Demux/2 -> Terminator1/1
  Demux/3 -> OATemp/1, Density/1, Hp/1

== system 6DoF_V8_2024a_FULLY_WORKING_FG/Subsystem1/NED to LAT//LONG  ==
  N : Inport
  E : Inport  Port=2
  D : Inport  Port=3
  Product : Product
  Product1 : Product
  Product2 : Product
  Sqrt : Sqrt
  Sum : Sum  Inputs=|+++
  r : Outport
  wires:
  Product2/1 -> Sum/3
  N/1 -> Product/1, Product/2
  D/1 -> Product2/1, Product2/2
  E/1 -> Product1/1, Product1/2
  Sqrt/1 -> r/1
  Product/1 -> Sum/1
  Product1/1 -> Sum/2
  Sum/1 -> Sqrt/1

== system 6DoF_V8_2024a_FULLY_WORKING_FG/Waypoint Calc/Altitude Hold Autopilot ==
  altitude : Inport
  altitude_cmd : Inport  Port=2
  R/C : Inport  Port=3
  Climb : Subsystem  TreatAsAtomicUnit=on
  Debug : Scope
  Debug1 : Scope  NumInputPorts=2
  Debug_h_err : Scope
  Descent : Subsystem  TreatAsAtomicUnit=on
  If : If  IfExpression=u1 < -100  ElseIfExpressions=u1 > 100
  Level : Subsystem  TreatAsAtomicUnit=on
  Merge : Merge  Inputs=3
  Merge1 : Merge  Inputs=3
  Sum1 : Sum  Inputs=+|-
  del_e_auto : Outport
  wires:
  altitude/1 -> Debug1/2, Sum1/1  "Altitude"
  altitude_cmd/1 -> Sum1/2
  If/1 -> Climb/Action
  If/2 -> Descent/Action
  If/3 -> Level/Action
  Sum1/1 -> Debug_h_err/1, Level/1(h_error), If/1
  Climb/1(del_e) -> Merge/1
  Descent/1(del_e) -> Merge/2
  Level/1(dele) -> Merge/3
  Merge/1 -> del_e_auto/1
  Climb/2(Debug) -> Merge1/1
  Descent/2(Debug) -> Merge1/2
  Level/2(debug) -> Merge1/3
  Merge1/1 -> Debug1/1, Debug/1  "Debug"
  R/C/1 -> Descent/1(R/C), Climb/1(R/C)

== system 6DoF_V8_2024a_FULLY_WORKING_FG/Waypoint Calc/Waypoint1 ==
  Range : Inport
  Counter : dspswit3/Counter  Direction=Up  CountEvent=Rising edge  CounterSize=User defined  MaxCount=255  InitialCount=1  Output=Count and Hit  HitValue=32  ResetInput=on  SamplesPerFrame=1  Ts=1  CntDtype=double  HitDtype=Logical
  Less Than : RelationalOperator  Operator=<  OutDataTypeStr=boolean  RndMeth=Simplest  InputSameDT=off
  Min range : Constant  Value=100
  Multiport Switch : MultiPortSwitch  Inputs=4  SaturateOnIntegerOverflow=off  InputSameDT=off
  Prevent Algebra shit from breaking : Memory
  Unit Delay : UnitDelay  SampleTime=-1  HasFrameUpgradeWarning=on
  WP1 : Constant  Value=WP1
  WP2 : Constant  Value=WP2
  WP3 : Constant  Value=WP3
  WP4 : Constant  Value=[0 100000 5000]
  Waypoint selected : Scope
  Waypoint Coords : Outport
  wires:
  Less Than/1 -> Unit Delay/1
  Min range/1 -> Less Than/2
  Range/1 -> Less Than/1
  Counter/1 -> Waypoint selected/1, Multiport Switch/1
  WP4/1 -> Multiport Switch/5
  Unit Delay/1 -> Counter/1
  WP3/1 -> Multiport Switch/4
  WP2/1 -> Multiport Switch/3
  WP1/1 -> Multiport Switch/2
  Multiport Switch/1 -> Waypoint Coords/1

== system 6DoF_V8_2024a_FULLY_WORKING_FG/Waypoint Calc/pi Bound1 ==
  In : Inport
  2pi : Constant  Value=2*pi
  Math Function : Math  Operator=mod  SignedPower=on
  Sum1 : Sum  Inputs=|+-  InputSameDT=on  SaturateOnIntegerOverflow=on  OutDataTypeStr=Inherit: Same as first input
  Sum2 : Sum  Inputs=|++  InputSameDT=on  SaturateOnIntegerOverflow=on  OutDataTypeStr=Inherit: Same as first input
  pi : Constant  Value=pi
  Out : Outport
  wires:
  Sum1/1 -> Out/1
  pi/1 -> Sum1/2, Sum2/2
  Sum2/1 -> Math Function/1
  In/1 -> Sum2/1
  2pi/1 -> Math Function/2
  Math Function/1 -> Sum1/1

== system 6DoF_V8_2024a_FULLY_WORKING_FG/Aircraft_Dynamics/Aerodynamics/Aero Forces and Moments ==
  dyn(q) : Inport
  CD : Inport  Port=2
  CY : Inport  Port=3
  CL : Inport  Port=4
  Wind Para : Inport  Port=5
  Croll : Inport  Port=6
  CM : Inport  Port=7
  CN : Inport  Port=8
  Aerodynamic Forces : Subsystem
  Aerodynamic Moments : Subsystem
  Faero : Outport
  Maero : Outport  Port=2
  wires:
  dyn(q)/1 -> Aerodynamic Moments/1(dyn(q)), Aerodynamic Forces/5(dyn(q))
  CD/1 -> Aerodynamic Forces/1(CD)
  CY/1 -> Aerodynamic Forces/2(CY)
  CL/1 -> Aerodynamic Forces/3(CL)
  Wind Para/1 -> Aerodynamic Forces/4(Wind Para)
  Croll/1 -> Aerodynamic Moments/2(Croll)
  CM/1 -> Aerodynamic Moments/3(CM)
  CN/1 -> Aerodynamic Moments/4(CN)
  Aerodynamic Forces/1(FaeroBody) -> Faero/1
  Aerodynamic Moments/1(Maero) -> Maero/1

== system 6DoF_V8_2024a_FULLY_WORKING_FG/Aircraft_Dynamics/Aerodynamics/CD ==
  Wind Parameters : Inport
  Controls : Inport  Port=2
  Mach No. : Inport  Port=3
  "   1" : Terminator
  "   6" : Terminator
  Get Alpha : Subsystem
  Math Function : Math  Operator=square  SignedPower=on
  Sum : Sum  SaturateOnIntegerOverflow=on
  cda2 : Gain  Gain=cda2  SaturateOnIntegerOverflow=on  OutDataTypeStr=Inherit: Same as input  ParamDataTypeStr=Inherit: Same as input
  cdo : Constant  Value=cdo
  CD : Outport
  wires:
  Wind Parameters/1 -> Get Alpha/1(windPar)
  Sum/1 -> CD/1
  Controls/1 -> "   6"/1
  Get Alpha/1(Alpha) -> Math Function/1
  Math Function/1 -> cda2/1
  cda2/1 -> Sum/2
  Mach No./1 -> "   1"/1
  cdo/1 -> Sum/1

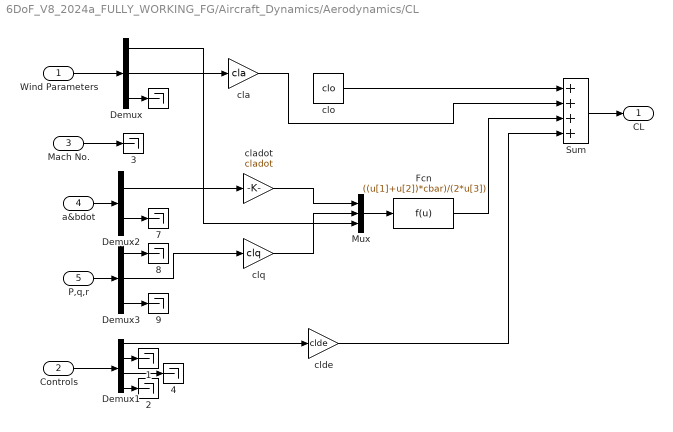
== system 6DoF_V8_2024a_FULLY_WORKING_FG/Aircraft_Dynamics/Aerodynamics/CL ==
  Wind Parameters : Inport
  Controls : Inport  Port=2
  Mach No. : Inport  Port=3
  a&bdot : Inport  Port=4
  P,q,r : Inport  Port=5
     {,1..4,7..9} (8 alike) : Terminator
  Demux : Demux  Outputs=3
      settings: DisplayOption=none
  Demux1 : Demux
      settings: DisplayOption=none
  Demux2 : Demux  Outputs=2
      settings: DisplayOption=none
  Demux3 : Demux  Outputs=3
      settings: DisplayOption=none
  Fcn : Fcn  Expr=((u[1]+u[2])*cbar)/(2*u[3])
  Mux : Mux  Inputs=3
  Sum : Sum  Inputs=++++  SaturateOnIntegerOverflow=on
  cla : Gain  Gain=cla  SaturateOnIntegerOverflow=on  OutDataTypeStr=Inherit: Same as input  ParamDataTypeStr=Inherit: Same as input
  cladot : Gain  Gain=cladot  SaturateOnIntegerOverflow=on  OutDataTypeStr=Inherit: Same as input  ParamDataTypeStr=Inherit: Same as input
  clde : Gain  Gain=clde  SaturateOnIntegerOverflow=on  OutDataTypeStr=Inherit: Same as input  ParamDataTypeStr=Inherit: Same as input
  clo : Constant  Value=clo
  clq : Gain  Gain=clq  SaturateOnIntegerOverflow=on  OutDataTypeStr=Inherit: Same as input  ParamDataTypeStr=Inherit: Same as input
  CL : Outport
  wires:
  Mux/1 -> Fcn/1
  Demux/1 -> Mux/3
  clo/1 -> Sum/1
  Demux2/2 -> "   7"/1
  Demux3/1 -> "   8"/1
  Demux3/3 -> "   9"/1
  Wind Parameters/1 -> Demux/1
  Sum/1 -> CL/1
  Controls/1 -> Demux1/1
  a&bdot/1 -> Demux2/1
  P,q,r/1 -> Demux3/1
  Demux/3 -> "   "/1
  Demux1/4 -> "   2"/1
  cla/1 -> Sum/2
  Demux2/1 -> cladot/1
  cladot/1 -> Mux/1
  Demux/2 -> cla/1
  clq/1 -> Mux/2
  Mach No./1 -> "   3"/1
  Demux3/2 -> clq/1
  Demux1/1 -> clde/1
  Demux1/2 -> "   1"/1
  Demux1/3 -> "   4"/1
  Fcn/1 -> Sum/3
  clde/1 -> Sum/4

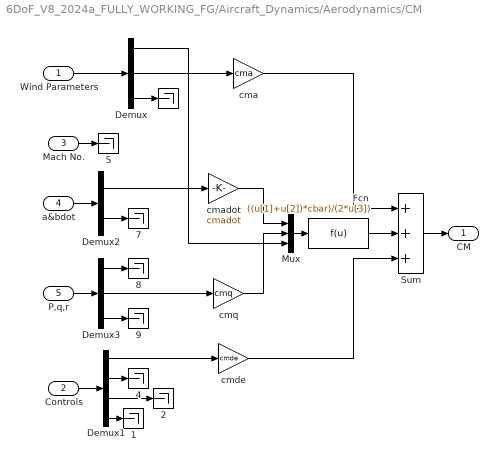
== system 6DoF_V8_2024a_FULLY_WORKING_FG/Aircraft_Dynamics/Aerodynamics/CM ==
  Wind Parameters : Inport
  Controls : Inport  Port=2
  Mach No. : Inport  Port=3
  a&bdot : Inport  Port=4
  P,q,r : Inport  Port=5
     {,1..2,4..5,7..9} (8 alike) : Terminator
  Demux : Demux  Outputs=3
      settings: DisplayOption=none
  Demux1 : Demux
      settings: DisplayOption=none
  Demux2 : Demux  Outputs=2
      settings: DisplayOption=none
  Demux3 : Demux  Outputs=3
      settings: DisplayOption=none
  Fcn : Fcn  Expr=((u[1]+u[2])*cbar)/(2*u[3])
  Mux : Mux  Inputs=3
  Sum : Sum  Inputs=+++  SaturateOnIntegerOverflow=on
  cma : Gain  Gain=cma  SaturateOnIntegerOverflow=on  OutDataTypeStr=Inherit: Same as input  ParamDataTypeStr=Inherit: Same as input
  cmadot : Gain  Gain=cmadot  SaturateOnIntegerOverflow=on  OutDataTypeStr=Inherit: Same as input  ParamDataTypeStr=Inherit: Same as input
  cmde : Gain  Gain=cmde  SaturateOnIntegerOverflow=on  OutDataTypeStr=Inherit: Same as input  ParamDataTypeStr=Inherit: Same as input
  cmq : Gain  Gain=cmq  SaturateOnIntegerOverflow=on  OutDataTypeStr=Inherit: Same as input  ParamDataTypeStr=Inherit: Same as input
  CM : Outport
  wires:
  Demux2/2 -> "   7"/1
  Demux3/1 -> "   8"/1
  Demux3/3 -> "   9"/1
  Wind Parameters/1 -> Demux/1
  Sum/1 -> CM/1
  Controls/1 -> Demux1/1
  a&bdot/1 -> Demux2/1
  P,q,r/1 -> Demux3/1
  Demux/3 -> "   "/1
  Demux1/4 -> "   1"/1
  Demux1/3 -> "   2"/1
  Demux/2 -> cma/1
  cmadot/1 -> Mux/1
  cmq/1 -> Mux/2
  Mux/1 -> Fcn/1
  Demux1/2 -> "   4"/1
  Mach No./1 -> "   5"/1
  Demux/1 -> Mux/3
  cma/1 -> Sum/1
  Demux1/1 -> cmde/1
  Demux2/1 -> cmadot/1
  Demux3/2 -> cmq/1
  Fcn/1 -> Sum/2
  cmde/1 -> Sum/3

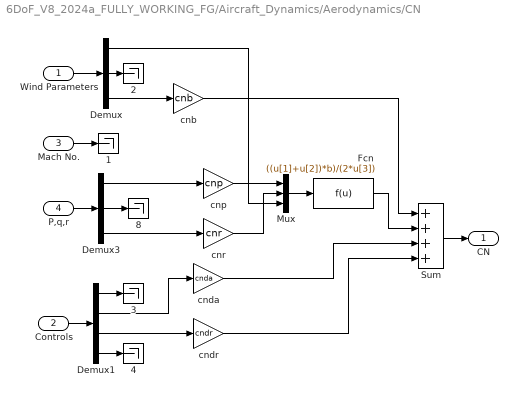
== system 6DoF_V8_2024a_FULLY_WORKING_FG/Aircraft_Dynamics/Aerodynamics/CN ==
  Wind Parameters : Inport
  Controls : Inport  Port=2
  Mach No. : Inport  Port=3
  P,q,r : Inport  Port=4
     {1..4,8} (5 alike) : Terminator
  Demux : Demux  Outputs=3
      settings: DisplayOption=none
  Demux1 : Demux
      settings: DisplayOption=none
  Demux3 : Demux  Outputs=3
      settings: DisplayOption=none
  Fcn : Fcn  Expr=((u[1]+u[2])*b)/(2*u[3])
  Mux : Mux  Inputs=3
  Sum : Sum  Inputs=++++  SaturateOnIntegerOverflow=on
  cnb : Gain  Gain=cnb  SaturateOnIntegerOverflow=on  OutDataTypeStr=Inherit: Same as input  ParamDataTypeStr=Inherit: Same as input
  cnda : Gain  Gain=cnda  SaturateOnIntegerOverflow=on  OutDataTypeStr=Inherit: Same as input  ParamDataTypeStr=Inherit: Same as input
  cndr : Gain  Gain=cndr  SaturateOnIntegerOverflow=on  OutDataTypeStr=Inherit: Same as input  ParamDataTypeStr=Inherit: Same as input
  cnp : Gain  Gain=cnp  SaturateOnIntegerOverflow=on  OutDataTypeStr=Inherit: Same as input  ParamDataTypeStr=Inherit: Same as input
  cnr : Gain  Gain=cnr  SaturateOnIntegerOverflow=on  OutDataTypeStr=Inherit: Same as input  ParamDataTypeStr=Inherit: Same as input
  CN : Outport
  wires:
  Mux/1 -> Fcn/1
  Demux/2 -> "   2"/1
  Wind Parameters/1 -> Demux/1
  Sum/1 -> CN/1
  Controls/1 -> Demux1/1
  P,q,r/1 -> Demux3/1
  Demux3/2 -> "   8"/1
  cnb/1 -> Sum/1
  Mach No./1 -> "   1"/1
  Demux/3 -> cnb/1
  Demux/1 -> Mux/3
  Demux3/1 -> cnp/1
  cnp/1 -> Mux/1
  Demux3/3 -> cnr/1
  cnr/1 -> Mux/2
  Demux1/2 -> cnda/1
  Demux1/3 -> cndr/1
  Fcn/1 -> Sum/2
  cnda/1 -> Sum/3
  cndr/1 -> Sum/4
  Demux1/1 -> "   3"/1
  Demux1/4 -> "   4"/1

== system 6DoF_V8_2024a_FULLY_WORKING_FG/Aircraft_Dynamics/Aerodynamics/CY ==
  Wind Parameters : Inport
  Controls : Inport  Port=2
  Mach No. : Inport  Port=3
  P,q,r : Inport  Port=4
     {2,7..12} (7 alike) : Terminator
  Demux : Demux  Outputs=3
      settings: DisplayOption=none
  Demux1 : Demux
      settings: DisplayOption=none
  Sum : Sum  SaturateOnIntegerOverflow=on
  cyb : Gain  Gain=cyb  SaturateOnIntegerOverflow=on  OutDataTypeStr=Inherit: Same as input  ParamDataTypeStr=Inherit: Same as input
  cydr : Gain  Gain=cydr  SaturateOnIntegerOverflow=on  OutDataTypeStr=Inherit: Same as input  ParamDataTypeStr=Inherit: Same as input
  CY : Outport
  wires:
  Demux/2 -> "   9"/1
  Wind Parameters/1 -> Demux/1
  Sum/1 -> CY/1
  Controls/1 -> Demux1/1
  P,q,r/1 -> "   8"/1
  Demux/3 -> cyb/1
  Mach No./1 -> "   2"/1
  Demux1/3 -> cydr/1
  Demux1/1 -> "   10"/1
  Demux1/2 -> "   7"/1
  Demux1/4 -> "   11"/1
  cyb/1 -> Sum/1
  cydr/1 -> Sum/2
  Demux/1 -> "   12"/1

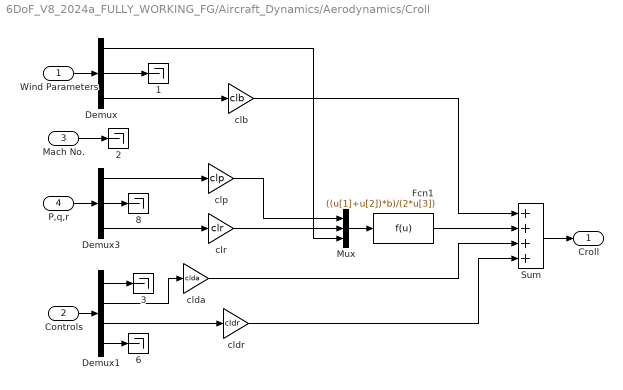
== system 6DoF_V8_2024a_FULLY_WORKING_FG/Aircraft_Dynamics/Aerodynamics/Croll ==
  Wind Parameters : Inport
  Controls : Inport  Port=2
  Mach No. : Inport  Port=3
  P,q,r : Inport  Port=4
     {1..3,6,8} (5 alike) : Terminator
  Demux : Demux  Outputs=3
      settings: DisplayOption=none
  Demux1 : Demux
      settings: DisplayOption=none
  Demux3 : Demux  Outputs=3
      settings: DisplayOption=none
  Fcn1 : Fcn  Expr=((u[1]+u[2])*b)/(2*u[3])
  Mux : Mux  Inputs=3
  Sum : Sum  Inputs=++++  SaturateOnIntegerOverflow=on
  clb : Gain  Gain=clb  SaturateOnIntegerOverflow=on  OutDataTypeStr=Inherit: Same as input  ParamDataTypeStr=Inherit: Same as input
  clda : Gain  Gain=clda  SaturateOnIntegerOverflow=on  OutDataTypeStr=Inherit: Same as input  ParamDataTypeStr=Inherit: Same as input
  cldr : Gain  Gain=cldr  SaturateOnIntegerOverflow=on  OutDataTypeStr=Inherit: Same as input  ParamDataTypeStr=Inherit: Same as input
  clp : Gain  Gain=clp  SaturateOnIntegerOverflow=on  OutDataTypeStr=Inherit: Same as input  ParamDataTypeStr=Inherit: Same as input
  clr : Gain  Gain=clr  SaturateOnIntegerOverflow=on  OutDataTypeStr=Inherit: Same as input  ParamDataTypeStr=Inherit: Same as input
  Croll : Outport
  wires:
  Mux/1 -> Fcn1/1
  Demux/2 -> "   1"/1
  Wind Parameters/1 -> Demux/1
  Sum/1 -> Croll/1
  Controls/1 -> Demux1/1
  P,q,r/1 -> Demux3/1
  Demux3/2 -> "   8"/1
  Demux1/1 -> "   3"/1
  clp/1 -> Mux/1
  clb/1 -> Sum/1
  Demux/1 -> Mux/3
  Demux/3 -> clb/1
  Mach No./1 -> "   2"/1
  Demux3/1 -> clp/1
  Fcn1/1 -> Sum/2
  Demux3/3 -> clr/1
  clr/1 -> Mux/2
  Demux1/4 -> "   6"/1
  Demux1/2 -> clda/1
  Demux1/3 -> cldr/1
  clda/1 -> Sum/3
  cldr/1 -> Sum/4

== system 6DoF_V8_2024a_FULLY_WORKING_FG/Aircraft_Dynamics/Equations of motion numerical integration /Flat Earth Navigation ==
  note: 1  roll
      | 2  pitch
      | 3  yaw
      | 4 u
      | 5 v
      | 6 w
  Euler Angles : Inport
  Velocity : Inport  Port=2
  Alt : Integrator  InitialCondition=initalt
  Alttitude Dot : Fcn  Expr=u[4] * sin(u[2]) - u[5] * sin(u[1]) * cos(u[2]) - u[6] * cos(u[1]) * cos(u[2])
  Demux : Demux  Outputs=3
      settings: DisplayOption=none
  Demux1 : Demux  Outputs=3
      settings: DisplayOption=none
  East : Integrator  InitialCondition=initeast
  East Dot : Fcn  Expr=u[4] * cos(u[2])* sin(u[3]) + u[5] * (cos(u[1])*cos(u[3]) + sin(u[1])*sin(u[2])*sin(u[3])) + u[6] * (-sin(u[1])*cos(u[3])+cos(u[1])*sin(u[2])*sin(u[3]))
  Mux : Mux  Inputs=6
  Mux1 : Mux  Inputs=3
  North : Integrator  InitialCondition=initnorth
  North Dot : Fcn  Expr=u[4] * cos(u[2]) * cos(u[3]) + u[5]*(-cos(u[1])*sin(u[3])+sin(u[1])*sin(u[2])*sin(u[3]))+u[6]*(sin(u[1])*sin(u[3])+cos(u[1])*sin(u[2])*cos(u[3]))
  Position : Outport
  R/C : Outport  Port=2
  wires:
  Euler Angles/1 -> Demux/1
  Velocity/1 -> Demux1/1
  Demux/1 -> Mux/1
  Demux/2 -> Mux/2
  Demux/3 -> Mux/3
  Demux1/1 -> Mux/4
  Demux1/2 -> Mux/5
  Demux1/3 -> Mux/6
  Mux/1 -> East Dot/1, Alttitude Dot/1, North Dot/1
  East Dot/1 -> East/1
  North Dot/1 -> North/1
  Alttitude Dot/1 -> R/C/1, Alt/1
  East/1 -> Mux1/2
  North/1 -> Mux1/1
  Alt/1 -> Mux1/3
  Mux1/1 -> Position/1

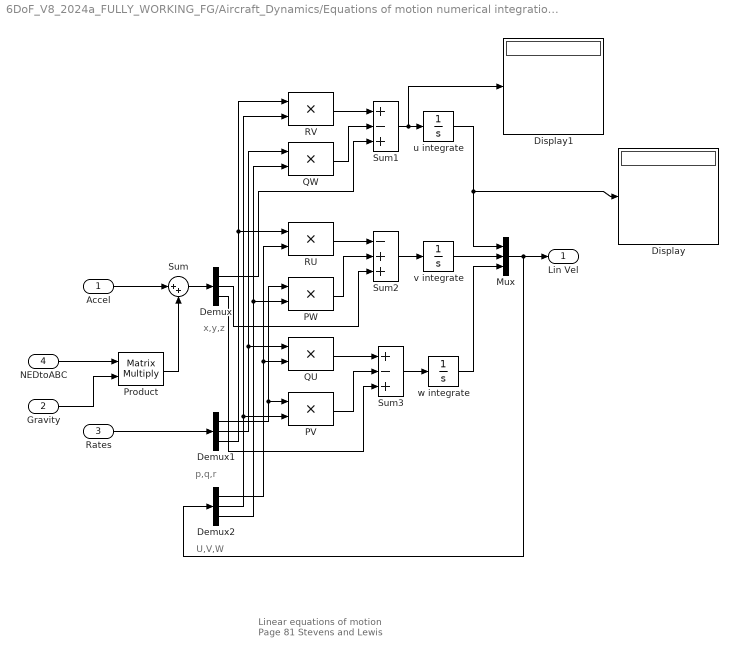
== system 6DoF_V8_2024a_FULLY_WORKING_FG/Aircraft_Dynamics/Equations of motion numerical integration /Force Equations ==
  note: U,V,W
  note: p,q,r
  note: x,y,z
  note: Linear equations of motion
      | Page 81 Stevens and Lewis
  Accel : Inport
  Gravity : Inport  Port=2
  Rates : Inport  Port=3
  NEDtoABC : Inport  Port=4
  Demux : Demux  Outputs=3
      settings: DisplayOption=none
  Demux1 : Demux  Outputs=3
      settings: DisplayOption=none
  Demux2 : Demux  Outputs=3
      settings: DisplayOption=none
  Display : Display
  Display1 : Display
  Mux : Mux  Inputs=3
  PV : Product  SaturateOnIntegerOverflow=on  OutDataTypeStr=Inherit: Same as first input
  PW : Product  SaturateOnIntegerOverflow=on  OutDataTypeStr=Inherit: Same as first input
  Product : Product  Multiplication=Matrix(*)  SaturateOnIntegerOverflow=on  OutDataTypeStr=Inherit: Same as first input
  QU : Product  SaturateOnIntegerOverflow=on  OutDataTypeStr=Inherit: Same as first input
  QW : Product  SaturateOnIntegerOverflow=on  OutDataTypeStr=Inherit: Same as first input
  RU : Product  SaturateOnIntegerOverflow=on  OutDataTypeStr=Inherit: Same as first input
  RV : Product  SaturateOnIntegerOverflow=on  OutDataTypeStr=Inherit: Same as first input
  Sum : Sum  Inputs=|++  SaturateOnIntegerOverflow=on
  Sum1 : Sum  Inputs=+-+  SaturateOnIntegerOverflow=on
  Sum2 : Sum  Inputs=-++  SaturateOnIntegerOverflow=on
  Sum3 : Sum  Inputs=+-+  SaturateOnIntegerOverflow=on
  u integrate : Integrator  InitialCondition=initu
  v integrate : Integrator  InitialCondition=initv
  w integrate : Integrator  InitialCondition=initw
  Lin Vel : Outport
  wires:
  Sum/1 -> Demux/1
  Accel/1 -> Sum/1
  Rates/1 -> Demux1/1
  Mux/1 -> Demux2/1, Lin Vel/1
  Demux1/3 -> RV/1, RU/1
  Demux2/2 -> RV/2, PV/2
  RV/1 -> Sum1/1
  Demux1/2 -> QW/1, QU/1
  Demux2/3 -> QW/2, PW/2
  QW/1 -> Sum1/2
  Demux/1 -> Sum1/3
  Demux2/1 -> RU/2, QU/2
  RU/1 -> Sum2/1
  Demux1/1 -> PV/1, PW/1
  PW/1 -> Sum2/2
  Demux/2 -> Sum2/3
  QU/1 -> Sum3/1
  PV/1 -> Sum3/2
  Demux/3 -> Sum3/3
  Gravity/1 -> Product/2
  NEDtoABC/1 -> Product/1
  Product/1 -> Sum/2
  Sum1/1 -> u integrate/1, Display1/1
  Sum2/1 -> v integrate/1
  Sum3/1 -> w integrate/1
  u integrate/1 -> Mux/1, Display/1
  v integrate/1 -> Mux/2
  w integrate/1 -> Mux/3
